simulink model "Vel_Ramp"  (R2022a)
settings: Solver=VariableStepAuto  StartTime=0.0  StopTime=10.0  RelTol=1e-3
settings Model: Creator=hp  LastModifiedBy=hp

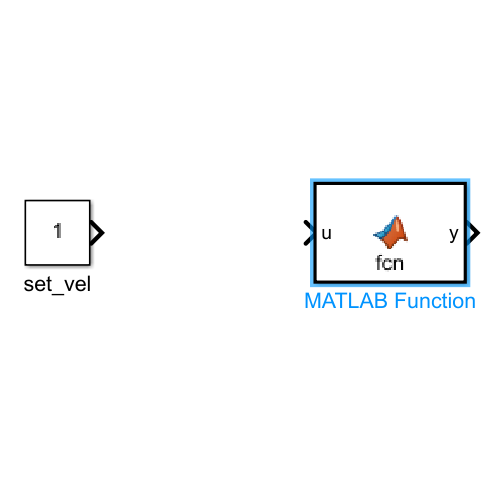
[thumbnail: Simulink's stored preview of the top-level diagram]
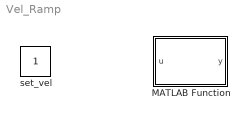
== system Vel_Ramp ==
  MATLAB Function : MATLAB Function  TreatAsAtomicUnit=on
  set_vel : Constant

== matlab function Vel_Ramp/MATLAB Function ==
  data: u input; y output
function y = fcn(u)

float max_step_size = abs(Ts*vel_ramp_rate);



y = u;
